simulink model "emldemo_sort"  (Simulink 7.6)
settings: Solver=FixedStepDiscrete  StartTime=0.0  StopTime=10.0  FixedStep=10  RelTol=1e-3
CloseFcn:
  | rtwprivate ssgencode ModelCloseRequest my_sort
settings Model: Creator=The MathWorks Inc.
settings OptimizationCC: InitFltsAndDblsToZero=on
settings DebuggingCC: SaveWithParameterizedLinksMsg=none  SignalResolutionControl=TryResolveAllWithWarning  MultiTaskDSMMsg=warning  MultiTaskCondExecSysMsg=none  StrictBusMsg=Warning
settings SFSimCC: SimCustomHeaderCode="#include \"c_sort.h\""  SimUserSources=c_sort.c  SimParseCustomCode=off
settings RTWCC: CustomInclude="#include \"c_sort.h\""  CustomSource=c_sort.c  IncludeERTFirstTime=on
settings GRTTargetCC: TargetFcnLib=ansi_tfl_tmw.mat

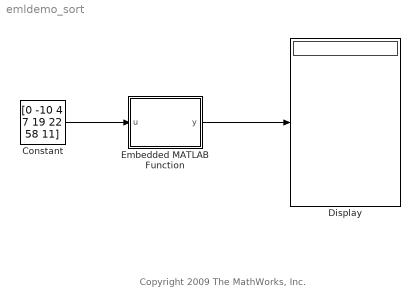
== system emldemo_sort ==
  note: Copyright 2009 The MathWorks, Inc.
  Constant : Constant  Value=[0 -10 4 7 19 22 58 11]
  Display : Display
  Embedded MATLAB Function : Stateflow chart  TreatAsAtomicUnit=on
  wires:
  Constant/1 -> Embedded MATLAB Function/1(u)
  Embedded MATLAB Function/1(y) -> Display/1

== matlab function Embedded MATLAB Function ==
  data: u input double; y output double
%#eml 
% The directive %#eml helps detect compile-time
% violations of Embedded MATLAB syntax and semantics
% in M-functions
function y = my_sort(u)

% Constrain 'y' to the same size and class as 'u'
y = u;

% Identify the MATLAB function 'disp' as an extrinsic function
eml.extrinsic('disp');

% Constrain the return type of function 'c_sort'
%   to a logical value
s = false;

% Call C function 'my_sort' with arguments:
%     eml.rref(y) - A read only reference to 'y'
%     eml.wref(y) - A write only reference to 'y'
%     numel(y)    - The number of elements of 'y' (or 'u')
s = eml.ceval('c_sort', eml.rref(y), eml.wref(y), int32(numel(y)));

if s % Already sorted
    disp('Already sorted.');
end
